simulink model "InternalADC"  (R2018b)
settings: Solver=FixedStepDiscrete  StartTime=0.0  StopTime=Inf  RelTol=1e-3  EnableMultiTasking=on
undefined symbols (not defined in the file or in its folder): Down, GPTRIP1SEL, GPTRIP2SEL, TZ1, TZ2, Up
libraries: idelinklib_common x72, c2837xDlib x39, c2802xlib x33, simulink x19, c280xlib x2, c2000lib x1
(part 1 of 4)
settings Model: ExtModeTrigDuration=8  Creator=ThinkPad  LastModifiedBy=ThinkPad
settings OptimizationCC: DefaultUnderspecifiedDataType=single  EnhancedBackFolding=on  PassReuseOutputArgsAs=Individual arguments  MaxStackSize=512  OptimizeBlockOrder=speed  DifferentSizesBufferReuse=on  OptimizationCustomize=off
settings DebuggingCC: ParameterTunabilityLossMsg=error
settings HardwareCC: ProdBitPerChar=16  ProdBitPerInt=16  ProdBitPerPointer=32  ProdBitPerSizeT=32  ProdBitPerPtrDiffT=32  ProdLargestAtomicInteger=Integer  ProdLargestAtomicFloat=None  ProdWordSize=16  ProdLongLongMode=on  ProdHWDeviceType=Texas Instruments->C2000
settings SFSimCC: MATLABDynamicMemAlloc=off
settings RTWCC: SystemTargetFile=ert.tlc  HardwareBoard=TI Delfino F2837xD  TemplateMakefile=ert_default_tmf  GenerateReport=on  Toolchain=Texas Instruments Code Composer Studio (C2000)  IncludeHyperlinkInReport=on  LaunchReport=on  GenerateTraceInfo=on  GenerateTraceReport=on  GenerateTraceReportSl=on  GenerateTraceReportSf=on  GenerateTraceReportEml=on
settings CodeAppCC: ForceParamTrailComments=on  IgnoreCustomStorageClasses=off  OperatorAnnotations=on  SimulinkDataObjDesc=on  SFDataObjDesc=on  InsertBlockDesc=on
settings ERTTargetCC: CodeReplacementLibrary=TI C28x

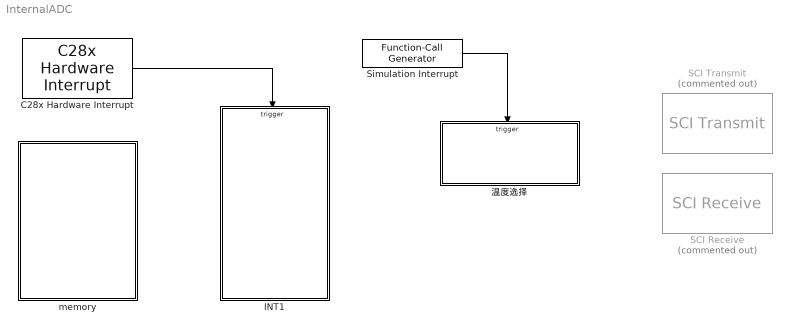
== system InternalADC ==
  C28x Hardware Interrupt : c2000lib/Scheduling/C28x Hardware Interrupt  irqnumbers=[3]  pienumbers=[1]  irqpriorities=[30]  irqpreempts=[0]  showinput=off  dspchiptype=C280X
      settings: SourceProductName=Embedded Coder Support Package for Texas Instruments C2000 Processors  SourceProductBaseCode=TIC2000
  INT1 : Subsystem
  SCI Receive : c280xlib/SCI Receive  Commented=on  sciModule=A  dataHead='S'  dataTail='E'  dataType=uint8  dataDim=1  initValue=0  errOption=Output the last received value  errValue=0  sampleTime=0.1  outputStatus=off  postInterrupt=off  numFifo=1
      settings: SourceProductName=Embedded Coder Support Package for Texas Instruments C2000 Processors  SourceProductBaseCode=TIC2000
  SCI Transmit : c280xlib/SCI Transmit  Commented=on  sciModule=A  dataHead='S'  dataTail='E'  postInterrupt=off  numFifo=1
      settings: SourceProductName=Embedded Coder Support Package for Texas Instruments C2000 Processors
  Simulation Interrupt : simulink/Ports & Subsystems/Function-Call Generator  sample_time=1  numberOfIterations=1
  memory : Subsystem
  温度选择 : Subsystem  TreatAsAtomicUnit=on
  wires:
  C28x Hardware Interrupt/1 -> INT1/Trigger
  Simulation Interrupt/1 -> 温度选择/Trigger

== system InternalADC/INT1 ==
  function : TriggerPort  TriggerType=function-call  VariantControl=(inherit)  SampleTime=1e-5
  ADC : Subsystem
  SPWM : Subsystem

== system InternalADC/memory ==
  A0 : idelinklib_common/Memory Allocate  variableName=A0  alignThisVariable=off  memoryAlignmentBoundary=4  dataType=int16  specifyQualifier=off  typeQualifier=volatile  dataDimension=1  specifyMemorySection=off  memorySection=A  bindMemorySection=on  sectionStartAddress=hex2dec('00081F00')  initializeMemory=off  initialValue=0
  A1 : idelinklib_common/Memory Allocate  variableName=A1  alignThisVariable=off  memoryAlignmentBoundary=4  dataType=int16  specifyQualifier=off  typeQualifier=volatile  dataDimension=1  specifyMemorySection=off  memorySection=A  bindMemorySection=on  sectionStartAddress=hex2dec('00081F00')  initializeMemory=off  initialValue=0
  A2 : idelinklib_common/Memory Allocate  variableName=A2  alignThisVariable=off  memoryAlignmentBoundary=4  dataType=int16  specifyQualifier=off  typeQualifier=volatile  dataDimension=1  specifyMemorySection=off  memorySection=A  bindMemorySection=on  sectionStartAddress=hex2dec('00081F00')  initializeMemory=off  initialValue=0
  A3 : idelinklib_common/Memory Allocate  variableName=A3  alignThisVariable=off  memoryAlignmentBoundary=4  dataType=int16  specifyQualifier=off  typeQualifier=volatile  dataDimension=1  specifyMemorySection=off  memorySection=A  bindMemorySection=on  sectionStartAddress=hex2dec('00081F00')  initializeMemory=off  initialValue=0
  A4 : idelinklib_common/Memory Allocate  variableName=A4  alignThisVariable=off  memoryAlignmentBoundary=4  dataType=int16  specifyQualifier=off  typeQualifier=volatile  dataDimension=1  specifyMemorySection=off  memorySection=A  bindMemorySection=on  sectionStartAddress=hex2dec('00081F00')  initializeMemory=on  initialValue=0
  A5 : idelinklib_common/Memory Allocate  variableName=A5  alignThisVariable=off  memoryAlignmentBoundary=4  dataType=int16  specifyQualifier=off  typeQualifier=volatile  dataDimension=1  specifyMemorySection=off  memorySection=A  bindMemorySection=on  sectionStartAddress=hex2dec('00081F00')  initializeMemory=off  initialValue=0
  B0 : idelinklib_common/Memory Allocate  variableName=B0  alignThisVariable=off  memoryAlignmentBoundary=4  dataType=int16  specifyQualifier=off  typeQualifier=volatile  dataDimension=1  specifyMemorySection=off  memorySection=A  bindMemorySection=on  sectionStartAddress=hex2dec('00081F00')  initializeMemory=off  initialValue=0
  B1 : idelinklib_common/Memory Allocate  variableName=B1  alignThisVariable=off  memoryAlignmentBoundary=4  dataType=int16  specifyQualifier=off  typeQualifier=volatile  dataDimension=1  specifyMemorySection=off  memorySection=A  bindMemorySection=on  sectionStartAddress=hex2dec('00081F00')  initializeMemory=off  initialValue=0
  B2 : idelinklib_common/Memory Allocate  variableName=B2  alignThisVariable=off  memoryAlignmentBoundary=4  dataType=int16  specifyQualifier=off  typeQualifier=volatile  dataDimension=1  specifyMemorySection=off  memorySection=A  bindMemorySection=on  sectionStartAddress=hex2dec('00081F00')  initializeMemory=off  initialValue=0
  B3 : idelinklib_common/Memory Allocate  variableName=B3  alignThisVariable=off  memoryAlignmentBoundary=4  dataType=int16  specifyQualifier=off  typeQualifier=volatile  dataDimension=1  specifyMemorySection=off  memorySection=A  bindMemorySection=on  sectionStartAddress=hex2dec('00081F00')  initializeMemory=off  initialValue=0
  B4 : idelinklib_common/Memory Allocate  variableName=B4  alignThisVariable=off  memoryAlignmentBoundary=4  dataType=int16  specifyQualifier=off  typeQualifier=volatile  dataDimension=1  specifyMemorySection=off  memorySection=A  bindMemorySection=on  sectionStartAddress=hex2dec('00081F00')  initializeMemory=on  initialValue=0
  B5 : idelinklib_common/Memory Allocate  variableName=B5  alignThisVariable=off  memoryAlignmentBoundary=4  dataType=int16  specifyQualifier=off  typeQualifier=volatile  dataDimension=1  specifyMemorySection=off  memorySection=A  bindMemorySection=on  sectionStartAddress=hex2dec('00081F00')  initializeMemory=off  initialValue=0
  C14 : idelinklib_common/Memory Allocate  variableName=C14  alignThisVariable=off  memoryAlignmentBoundary=4  dataType=int16  specifyQualifier=off  typeQualifier=volatile  dataDimension=1  specifyMemorySection=off  memorySection=A  bindMemorySection=on  sectionStartAddress=hex2dec('00081F00')  initializeMemory=off  initialValue=0
  C15 : idelinklib_common/Memory Allocate  variableName=C15  alignThisVariable=off  memoryAlignmentBoundary=4  dataType=int16  specifyQualifier=off  typeQualifier=volatile  dataDimension=1  specifyMemorySection=off  memorySection=A  bindMemorySection=on  sectionStartAddress=hex2dec('00081F00')  initializeMemory=off  initialValue=0
  C2 : idelinklib_common/Memory Allocate  variableName=C2  alignThisVariable=off  memoryAlignmentBoundary=4  dataType=int16  specifyQualifier=off  typeQualifier=volatile  dataDimension=1  specifyMemorySection=off  memorySection=A  bindMemorySection=on  sectionStartAddress=hex2dec('00081F00')  initializeMemory=off  initialValue=0
  C3 : idelinklib_common/Memory Allocate  variableName=C3  alignThisVariable=off  memoryAlignmentBoundary=4  dataType=int16  specifyQualifier=off  typeQualifier=volatile  dataDimension=1  specifyMemorySection=off  memorySection=A  bindMemorySection=on  sectionStartAddress=hex2dec('00081F00')  initializeMemory=off  initialValue=0
  C4 : idelinklib_common/Memory Allocate  variableName=C4  alignThisVariable=off  memoryAlignmentBoundary=4  dataType=int16  specifyQualifier=off  typeQualifier=volatile  dataDimension=1  specifyMemorySection=off  memorySection=A  bindMemorySection=on  sectionStartAddress=hex2dec('00081F00')  initializeMemory=off  initialValue=0
  C5 : idelinklib_common/Memory Allocate  variableName=C5  alignThisVariable=off  memoryAlignmentBoundary=4  dataType=int16  specifyQualifier=off  typeQualifier=volatile  dataDimension=1  specifyMemorySection=off  memorySection=A  bindMemorySection=on  sectionStartAddress=hex2dec('00081F00')  initializeMemory=off  initialValue=0
  D0 : idelinklib_common/Memory Allocate  variableName=D0  alignThisVariable=off  memoryAlignmentBoundary=4  dataType=int16  specifyQualifier=off  typeQualifier=volatile  dataDimension=1  specifyMemorySection=off  memorySection=A  bindMemorySection=on  sectionStartAddress=hex2dec('00081F00')  initializeMemory=off  initialValue=0
  D1 : idelinklib_common/Memory Allocate  variableName=D1  alignThisVariable=off  memoryAlignmentBoundary=4  dataType=int16  specifyQualifier=off  typeQualifier=volatile  dataDimension=1  specifyMemorySection=off  memorySection=A  bindMemorySection=on  sectionStartAddress=hex2dec('00081F00')  initializeMemory=off  initialValue=0
  D2 : idelinklib_common/Memory Allocate  variableName=D2  alignThisVariable=off  memoryAlignmentBoundary=4  dataType=int16  specifyQualifier=off  typeQualifier=volatile  dataDimension=1  specifyMemorySection=off  memorySection=A  bindMemorySection=on  sectionStartAddress=hex2dec('00081F00')  initializeMemory=off  initialValue=0
  D3 : idelinklib_common/Memory Allocate  variableName=D3  alignThisVariable=off  memoryAlignmentBoundary=4  dataType=int16  specifyQualifier=off  typeQualifier=volatile  dataDimension=1  specifyMemorySection=off  memorySection=A  bindMemorySection=on  sectionStartAddress=hex2dec('00081F00')  initializeMemory=off  initialValue=0
  D4 : idelinklib_common/Memory Allocate  variableName=D4  alignThisVariable=off  memoryAlignmentBoundary=4  dataType=int16  specifyQualifier=off  typeQualifier=volatile  dataDimension=1  specifyMemorySection=off  memorySection=A  bindMemorySection=on  sectionStartAddress=hex2dec('00081F00')  initializeMemory=on  initialValue=0
  D5 : idelinklib_common/Memory Allocate  variableName=D5  alignThisVariable=off  memoryAlignmentBoundary=4  dataType=int16  specifyQualifier=off  typeQualifier=volatile  dataDimension=1  specifyMemorySection=off  memorySection=A  bindMemorySection=on  sectionStartAddress=hex2dec('00081F00')  initializeMemory=off  initialValue=0

== system InternalADC/温度选择 ==
  function : TriggerPort  TriggerType=function-call  VariantControl=(inherit)
  000 : Subsystem
  001 : Subsystem
  010 : Subsystem
  011 : Subsystem
  100 : Subsystem
  101 : Subsystem
  110 : Subsystem
  111 : Subsystem
  Constant10 : Constant  OutDataTypeStr=uint16
  Demux : Demux  Outputs=3
  Integration 0 to maximal3 : Subsystem  mask{a=12}
      mask prompts: a "the maximal y"
  Multiport Switch : MultiPortSwitch  Inputs=8  DataPortForDefault=Additional data port  OutDataTypeStr=uint16
  Subsystem : Subsystem
  Terminator4 : Terminator
  wires:
  Constant10/1 -> Integration 0 to maximal3/1(x)
  Integration 0 to maximal3/1(y) -> Multiport Switch/1
  Multiport Switch/1 -> Demux/1
  Integration 0 to maximal3/2(Zero Trig) -> Terminator4/1
  Demux/1 -> Subsystem/1(S2)
  Demux/2 -> Subsystem/2(S1)
  Demux/3 -> Subsystem/3(S0)
  000/1(Out1) -> Multiport Switch/2
  001/1(Out1) -> Multiport Switch/3
  010/1(Out1) -> Multiport Switch/4
  011/1(Out1) -> Multiport Switch/5
  111/1(Out1) -> Multiport Switch/9
  110/1(Out1) -> Multiport Switch/8
  101/1(Out1) -> Multiport Switch/7
  100/1(Out1) -> Multiport Switch/6
